simulink library "tqd"  (R2021b)
settings: Solver=VariableStepAuto  StartTime=0.0  StopTime=10.0  RelTol=1e-3
undefined symbols (not defined in the file): ATQD_AfterTqMinGain_X_Deg, ATQD_APSCreepBaseTqD_X_kph, ATQD_APSCreepBaseTqD_Y_Deg, ATQD_APSCreepBaseTqR_X_kph, ATQD_APSCreepBaseTqR_Y_Deg, ATQD_APSCreepIterm_X_kph, ATQD_APSCreepIterm_Y_kph, ATQD_APSCreepPterm_X_kph, ATQD_APSCreepPterm_Y_kph, ATQD_APSDecReq_X_kph, ATQD_APSDecReq_Y_mps2, ATQD_APSDecReqCMD_X_kph, ATQD_APSDecReqTs_X_pct, ATQD_APSDecTimeGain_X_Deg, ATQD_APSDecTimeGain_Y_s, ATQD_APSReqLowSpd_X_Deg, ATQD_AutoHoldReleaseBPS_X_Deg, ATQD_AWDLoadTrqnsGain_X_kg, ATQD_AWDLoadTrqnsGain_Y_pct, ATQD_BOSEnBPSPosn_X_kph, ATQD_BOSMap_X_rpm, ATQD_BOSMap_Y_pct, ATQD_CreepBaseTqD_X_kph, ATQD_CreepBaseTqD_Y_Deg, ATQD_CreepBaseTqR_X_kph, ATQD_CreepBaseTqR_Y_Deg, ATQD_CreepBPSDisPosn_X_Deg, ATQD_CreepBPSDisPosnR_X_Deg, ATQD_CreepBPSEnPosn_X_Deg, ATQD_CreepBPSEnPosnR_X_Deg, ATQD_CreepDeltaTq_X_kph, ATQD_CreepIterm_X_kph, ATQD_CreepIterm_Y_kph, ATQD_CreepItermMaxLimit_X_pct, ATQD_CreepPreloadTime_X_kph, ATQD_CreepPreloadTq_X_kph, ATQD_CreepPreloadTq_Y_s, ATQD_CreepProtTq_X_Deg, ATQD_CreepPterm_X_kph, ATQD_CreepPterm_Y_kph, ATQD_CreepRrTqSpRat_X_rpm, ATQD_CreepRrTqSpRat_Y_Nm, ATQD_CreepTargetSpdD_X_pct, ATQD_CreepTargetSpdR_X_pct, ATQD_ECOTqMapD_X_rpm, ATQD_ECOTqMapD_Y_pct, ATQD_EMTqMapD_X_rpm, ATQD_EMTqMapD_Y_pct, ATQD_EOPDTqMapDCon_X_rpm, ATQD_EOPDTqMapDCon_Y_Deg, ATQD_EscapeModePedTq_X_pct, ATQD_EscapeModePedTq_Y_rpm, ATQD_EscapeModePedTqFr_X_pct, ATQD_EscapeModePedTqFr_Y_rpm, ATQD_EstInitVehWeight_X_c, ATQD_FAfterTqCMDGain_X_rpm, ATQD_FAfterTqCMDGain_Y_pct, ATQD_FrLossMAPLowV_X_rpm, ATQD_FrLossMAPLowV_Y_Nm, ATQD_FrMotActReduce_X_rpm ... (+772)
libraries: simulink x211, hcu_lib x179, tqr x3
(part 15 of 28)

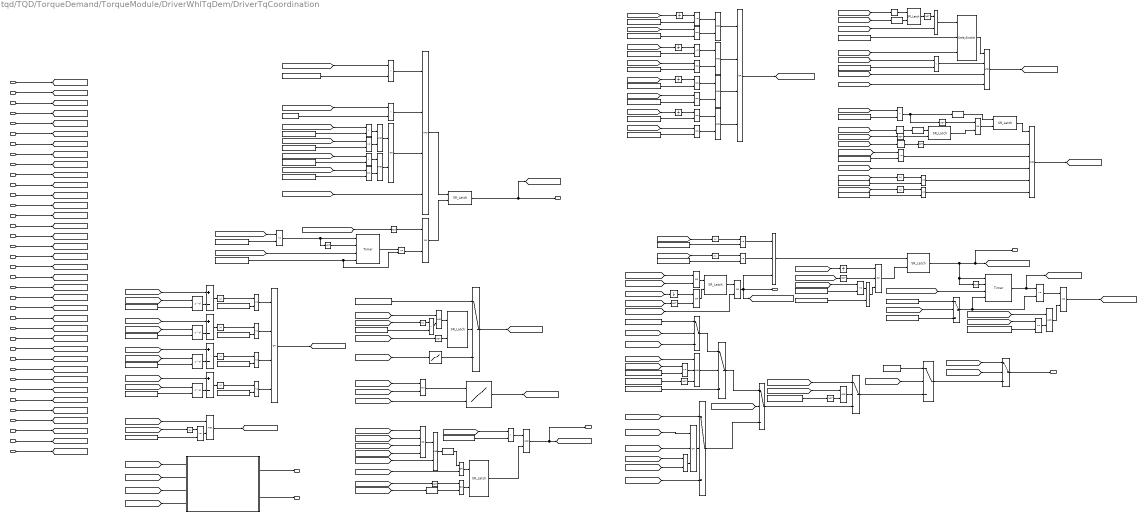
== system tqd/TQD/TorqueDemand/TorqueModule/DriverWhlTqDem/DriverTqCoordination ==
  VTQD_PedalMapWhlTq_Nm : Inport
  VTQD_CreepPrLoadEnable_flg : Inport  Port=2
  VTQD_CreepWhlTqDem_Nm : Inport  Port=3
  VTQD_BOSEnable_flg : Inport  Port=4
  VTQD_BOSTq_Nm : Inport  Port=5
  VVMC_LongAcc_Gps : Inport  Port=6
  VINP_VehSpeed_kph : Inport  Port=7
  VTQD_BrkSwSta_flg : Inport  Port=8
  VTQD_ActBPSPosn_pct : Inport  Port=9
  VTQD_LowIdleAccPedal_flg : Inport  Port=10
  VTQD_GearActualPosn_enum : Inport  Port=11
  task_time_s : Inport  Port=12
  VINP_FrEDURealTMTq_Nm : Inport  Port=13
  VINP_RrEDURealTMTq_Nm : Inport  Port=14
  VVMC_APSActive_flg : Inport  Port=15
  VVMC_ADASActive_flg : Inport  Port=16
  VINP_ACCVehHoldReq_flg : Inport  Port=17
  VTQD_CreepProtTqEn_flg : Inport  Port=18
  VTQD_TqTargetShaftSpd_rpm : Inport  Port=19
  VTQD_VehActSpd_kph : Inport  Port=20
  VTQD_APSReqTimer_s : Inport  Port=21
  VTQD_CreepEnable_flg : Inport  Port=22
  VTQR_RShaftSpdTqLimLow_flg : Inport  Port=23
  VTQR_RTimerTqLimLow_flg : Inport  Port=24
  VTQR_FShaftSpdTqLimLow_flg : Inport  Port=25
  VTQR_FTimerTqLimLow_flg : Inport  Port=26
  VTQD_ActAPSPosn_pct : Inport  Port=27
  VTQD_IVIRockModeEn_flg : Inport  Port=28
  VINP_LFRawWhlSpeed_kph : Inport  Port=29
  VINP_LRRawWhlSpeed_kph : Inport  Port=30
  VINP_RFRawWhlSpeed_kph : Inport  Port=31
  VINP_RRRawWhlSpeed_kph : Inport  Port=32
  VTQD_FrShaftSpd_rpm : Inport  Port=33
  VTQD_RrShaftSpd_rpm : Inport  Port=34
  VINP_ADASAEBSta_enum : Inport  Port=35
  VTQD_ActWhlSkipSta_enum : Inport  Port=36
  VDDM_VehMalfunLevel_enum : Inport  Port=37
  AND : Logic  Inputs=3  AllPortsSameDT=off  OutDataTypeStr=boolean
  AND{1..3,7..17} (14 alike) : Logic  AllPortsSameDT=off  OutDataTypeStr=boolean
  AND4 : Logic  Inputs=6  AllPortsSameDT=off  OutDataTypeStr=boolean
  AND5 : Logic  Inputs=4  AllPortsSameDT=off  OutDataTypeStr=boolean
  AND6 : Logic  Inputs=4  AllPortsSameDT=off  OutDataTypeStr=boolean
  Abs{,1..9} (10 alike) : Abs
  Add{,1..3} (4 alike) : Sum  Inputs=+-
  Constant : Constant  Value=KTQD_LoSpdCtrlBrkPos_pct
  Constant1 : Constant  Value=KTQD_RrPreLoadBoundary_Nm
  Constant{2,10,15,17} (4 alike) : Constant  Value=ZERO_FLOAT
  Constant11 : Constant  Value=KTQD_ADASHoldPreLoadspd_kph
  Constant12 : Constant  Value=KTQD_ADASHoldDelayEnTime_s
  Constant13 : Constant  Value=KTQD_EmergBrkSpd_kph
  Constant14 : Constant  Value=KTQD_EmergBrkLongAccel_Gps
  Constant16 : Constant  Value=KTQD_PreLoadTqHold_rpm
  Constant18 : Constant  Value=KTQD_OPDHoldPreLoadTime_s
  Constant19 : Constant  Value=KTQD_PreLoad_Holdtime_s
  Constant20 : Constant  Value=KTQD_APSZeroSpd_kph
  Constant21 : Constant  Value=ENUM_GEARACTUALPOSN_D
  Constant22 : Constant  Value=ENUM_GEARACTUALPOSN_D
  Constant{4,6,23..24} (4 alike) : Constant  Value=ENUM_GEARACTUALPOSN_R
  Constant25 : Constant  Value=KTQD_LoSPdBrkRlsTime_s
  Constant26 : Constant  Value=KTQD_LoSpdBrkRlsSpd_kph
  Constant27 : Constant  Value=KTQD_OPDHoldPreLoadBound_Nm
  Constant28 : Constant  Value=KTQD_OPDHoldPreLoadBound_Nm
  Constant29 : Constant  Value=KTQD_PreLoadDisSpd_kph
  Constant3 : Constant  Value=KTQD_RrPreLoadBoundary_Nm
  Constant{30,32,34,36} (4 alike) : Constant  Value=KTQD_EscModeWhlSpdDely_cnt
  Constant{31,33,35,37} (4 alike) : Constant  Value=KTQD_EscModeTqLimSpdDev_kph
  Constant38 : Constant  Value=KTQD_EscModeTqLimAccCon_Gps
  Constant39 : Constant  Value=KTQD_ESCModeTqCtrlSW_flg
  Constant40 : Constant  Value=ENUM_ADASAEBSTA_ACTIVE
  Constant41 : Constant  Value=KTQD_AEBEmergBrkSpd_kph
  Constant42 : Constant  Value=KTQD_APSPreLoadHoldtime_s
  Constant43 : Constant  Value=KTQD_RockModeWhlSkipSta_enum
  Constant44 : Constant  Value=KTQD_NewPrelaodSW_flg
  Constant45 : Constant  Value=ENUM_VEHMALFUNLEVEL_LEVEL3
  Constant5 : Constant  Value=ENUM_GEARACTUALPOSN_N
  Constant7 : Constant  Value=ENUM_GEARACTUALPOSN_P
  Constant8 : Constant  Value=ENUM_GEARACTUALPOSN_P
  Constant9 : Constant  Value=KTQD_PreLoadTq_Nm
  Constant96 : Constant  Value=KTQD_FailsafeActiveSW_flg
  Delay : Delay  DelayLength=1
  Delay1 : Delay  DelayLength=1
  Delay2 : Delay  DelayLength=1
  Delay{3..6} (4 alike) : Delay  DelayLengthSource=Input port
      settings: InputPortMap=u0,p1
  DelayEnable : hcu_lib/Basic_Blocks/DelayEnable
  Detect Change : simulink/Logic and Bit Operations/Detect Change  vinit=0  OutDataTypeStr=boolean
  Detect Decrease : simulink/Logic and Bit Operations/Detect Decrease  vinit=0.0  OutDataTypeStr=boolean
  Detect Increase : simulink/Logic and Bit Operations/Detect Increase  vinit=0.0  OutDataTypeStr=boolean
  Detect Increase1 : simulink/Logic and Bit Operations/Detect Increase  vinit=0.0  OutDataTypeStr=boolean
  Detect Increase2 : simulink/Logic and Bit Operations/Detect Increase  vinit=0.0  OutDataTypeStr=boolean
  Equal{1..4,6,8} (6 alike) : RelationalOperator  Operator===  OutDataTypeStr=boolean  RndMeth=Simplest
  Equal5 : RelationalOperator  Operator=~=  OutDataTypeStr=boolean  RndMeth=Simplest
  Equal7 : RelationalOperator  Operator=~=  OutDataTypeStr=boolean  RndMeth=Simplest
  Equal9 : RelationalOperator  Operator=~=  OutDataTypeStr=boolean  RndMeth=Simplest
  GreaterThan : RelationalOperator  OutDataTypeStr=boolean  RndMeth=Simplest
  Logical Operator : Logic  Inputs=3  AllPortsSameDT=off  OutDataTypeStr=boolean
  Logical Operator13 : Logic  AllPortsSameDT=off  OutDataTypeStr=boolean
  MTQD_EscapeModePedTq_Z_Nm : Lookup_n-D  BreakpointsForDimension1=ATQD_EscapeModePedTq_Y_rpm  BreakpointsForDimension2=ATQD_EscapeModePedTq_X_pct  Table=MTQD_EscapeModePedTq_Z_Nm  InternalRulePriority=Speed  RndMeth=Simplest  InputSameDT=on
      settings: InputPortMap=u0,u1
  MTQD_PreLoadTq_Y_Nm : Lookup_n-D  NumberOfTableDimensions=1  BreakpointsForDimension1=ATQD_PreLoadTq_X_s  Table=MTQD_PreLoadTq_Y_Nm  ExtrapMethod=Clip  InternalRulePriority=Speed  RndMeth=Simplest  InputSameDT=on
  Max : MinMax  Function=max  Inputs=2
  NOT{,1..12} (13 alike) : Logic  Operator=NOT  AllPortsSameDT=off  OutDataTypeStr=boolean
  New Preload Torque : Subsystem
  OR : Logic  Operator=OR  Inputs=3  AllPortsSameDT=off  OutDataTypeStr=boolean
  OR{2,4..8,10,12..13} (9 alike) : Logic  Operator=OR  AllPortsSameDT=off  OutDataTypeStr=boolean
  OR11 : Logic  Operator=OR  Inputs=4  AllPortsSameDT=off  OutDataTypeStr=boolean
  OR14 : Logic  Operator=OR  Inputs=3  AllPortsSameDT=off  OutDataTypeStr=boolean
  OR3 : Logic  Operator=OR  Inputs=4  AllPortsSameDT=off  OutDataTypeStr=boolean
  OR9 : Logic  Operator=OR  Inputs=4  AllPortsSameDT=off  OutDataTypeStr=boolean
  Relational Operator{,7,15..18,23} (7 alike) : RelationalOperator  OutDataTypeStr=boolean  RndMeth=Simplest
  Relational Operator{1..2,6,11..14,19} (8 alike) : RelationalOperator  Operator=<=  OutDataTypeStr=boolean  RndMeth=Simplest
  Relational Operator{3,8..10,21} (5 alike) : RelationalOperator  Operator=<  OutDataTypeStr=boolean  RndMeth=Simplest
  Relational Operator20 : RelationalOperator  Operator===  OutDataTypeStr=boolean  RndMeth=Simplest
  Relational Operator22 : RelationalOperator  Operator=>  OutDataTypeStr=boolean  RndMeth=Simplest
  Relational Operator4 : RelationalOperator  Operator=>  OutDataTypeStr=boolean  RndMeth=Simplest
  Relational Operator5 : RelationalOperator  Operator=>  OutDataTypeStr=boolean  RndMeth=Simplest
  SR_Latch{,1..7} (8 alike) : hcu_lib/Basic_Blocks/SR_Latch
  Switch{,1..4} (5 alike) : Switch  Criteria=u2 ~= 0
      Switch1 settings: AttributesFormatString=<%<Criteria>>
      Switch2 settings: AttributesFormatString=<%<Criteria>>
  Switch{5..8} (4 alike) : Switch  Criteria=u2 > Threshold
  Timer : hcu_lib/Basic_Blocks/Timer
  Timer1 : hcu_lib/Basic_Blocks/Timer
  Unit Delay{1..6} (6 alike) : UnitDelay  SampleTime=-1  HasFrameUpgradeWarning=on
  VTQD_DriverWhlTqDem_Nm : Outport
  VTQD_LoSpdBrkCtrl_flg : Outport  Port=2
  VTQD_PreLoadHold_flg : Outport  Port=3
  VTQD_PreLoadPreEn_flg : Outport  Port=4
  VTQD_EscapModeTqLim_flg : Outport  Port=5
  VTQD_FrPreloadTq_Nm : Outport  Port=6
  VTQD_RrPreloadTq_Nm : Outport  Port=7
  wires:
  VTQD_PedalMapWhlTq_Nm/1 -> [VTQD_PedalMapWhlTq_Nm]
  VTQD_CreepPrLoadEnable_flg/1 -> [VTQD_CreepPrLoadEnable_flg]
  VTQD_CreepWhlTqDem_Nm/1 -> [VTQD_CreepWhlTqDem_Nm]
  VTQD_BOSEnable_flg/1 -> [VTQD_BOSEnable_flg]
  VTQD_BOSTq_Nm/1 -> [VTQD_BOSTq_Nm]
  [VTQD_BOSEnable_flg] -> Switch1/2
  [VTQD_PedalMapWhlTq_Nm] -> Switch2/3
  [VTQD_CreepWhlTqDem_Nm] -> Switch2/1
  [VTQD_ActBPSPosn_pct] -> Relational Operator/1
  Constant/1 -> Relational Operator/2
  SR_Latch/1 -> [VTQD_LoSpdBrkCtrl_flg], VTQD_LoSpdBrkCtrl_flg/1  "VTQD_LoSpdBrkCtrl_flg"
  Constant10/1 -> Switch/1
  Switch1/1 -> VTQD_DriverWhlTqDem_Nm/1  "VTQD_DriverWhlTqDem_Nm"
  Switch/1 -> Switch1/3
  [VTQD_LowIdleAccPedal_flg] -> NOT/1
  [VTQD_VehActSpd_kph] -> Relational Operator6/1
  Constant26/1 -> Relational Operator6/2
  Relational Operator6/1 -> Timer/1, NOT1/1
  Timer/1 -> Relational Operator7/1
  NOT/1 -> OR2/1
  Relational Operator7/1 -> OR2/2
  OR2/1 -> SR_Latch/2  "VTQD_LoBrkCtrlReset_flg"
  NOT1/1 -> Timer/2
  Constant13/1 -> Relational Operator10/2
  [VINP_VehSpeed_kph] -> Relational Operator10/1
  Constant15/1 -> Relational Operator9/2
  Constant14/1 -> Relational Operator8/2
  [VVMC_LongAcc_Gps] -> Relational Operator8/1
  Relational Operator9/1 -> AND6/2
  Relational Operator8/1 -> AND6/1
  [task_time_s] -> Timer/3
  VVMC_LongAcc_Gps/1 -> [VVMC_LongAcc_Gps]
  VINP_VehSpeed_kph/1 -> [VINP_VehSpeed_kph]
  VTQD_BrkSwSta_flg/1 -> [VTQD_BrkSwSta_flg]
  VTQD_ActBPSPosn_pct/1 -> [VTQD_ActBPSPosn_pct]
  VTQD_LowIdleAccPedal_flg/1 -> [VTQD_LowIdleAccPedal_flg]
  VTQD_GearActualPosn_enum/1 -> [VTQD_GearActualPosn_enum]
  task_time_s/1 -> [task_time_s]
  Constant25/1 -> Relational Operator7/2, Timer/4
  AND6/1 -> SR_Latch/1  "VTQD_TestLoSpdBrkCtrl_flg"
  Timer1/1 -> [VTQD_PreLoadHoldtime_s], GreaterThan/1  "VTQD_PreLoadHoldtime_s"
  [VTQD_PreLoadPreEn_flg] -> Switch4/2
  [VTQD_HoldtimeEnd_flg] -> Unit Delay4/1
  [task_time_s] -> Timer1/3
  Unit Delay2/1 -> Equal5/1
  [VTQD_GearActualPosn_enum] -> Unit Delay2/1
  Constant23/1 -> Equal7/2
  [VTQD_GearActualPosn_enum] -> Equal8/1
  Equal5/1 -> AND8/1
  AND9/1 -> OR3/2
  Constant21/1 -> Equal5/2
  Constant24/1 -> Equal8/2
  Unit Delay3/1 -> Equal7/1
  Constant22/1 -> Equal6/2
  AND8/1 -> OR3/1
  [VTQD_GearActualPosn_enum] -> Unit Delay3/1
  [VTQD_GearActualPosn_enum] -> Equal6/1
  Equal6/1 -> AND8/2
  Equal8/1 -> AND9/2
  OR3/1 -> [VTQD_ShiftPreload_flg]  "VTQD_ShiftPreload_flg"
  Equal7/1 -> AND9/1
  NOT2/1 -> Timer1/2
  Unit Delay4/1 -> OR4/1
  OR4/1 -> SR_Latch1/2
  Switch2/1 -> Switch4/3
  [VTQD_LowIdleAccPedal_flg] -> NOT3/1
  NOT3/1 -> OR4/2
  [VTQD_LoSpdBrkCtrl_flg] -> Switch/2
  VINP_FrEDURealTMTq_Nm/1 -> [VINP_FrEDURealTMTq_Nm]
  VINP_RrEDURealTMTq_Nm/1 -> [VINP_RrEDURealTMTq_Nm]
  [VTQD_GearActualPosn_enum] -> Equal2/1
  Constant5/1 -> Equal2/2
  Equal2/1 -> AND1/2
  Equal1/1 -> AND1/1
  Constant4/1 -> Equal1/2
  AND1/1 -> OR3/3
  [VTQD_GearActualPosn_enum] -> Unit Delay1/1
  Unit Delay1/1 -> Equal1/1
  Constant3/1 -> Relational Operator2/2
  Relational Operator2/1 -> AND/1
  Constant1/1 -> Relational Operator1/2
  Abs1/1 -> Relational Operator2/1
  Relational Operator1/1 -> AND/2
  Abs/1 -> Relational Operator1/1
  [VINP_RrEDURealTMTq_Nm] -> Abs/1
  [VINP_FrEDURealTMTq_Nm] -> Abs1/1
  OR5/1 -> AND/3, VTQD_PreLoadPreEn_flg/1, [VTQD_PreLoadPreEn_flg]  "VTQD_PreLoadPreEn_flg"
  Switch3/1 -> Switch4/1
  Constant2/1 -> Switch3/3
  Unit Delay5/1 -> Equal3/1
  [VTQD_GearActualPosn_enum] -> Unit Delay5/1
  Constant6/1 -> Equal3/2
  Equal3/1 -> AND2/1
  Equal4/1 -> AND2/2
  Constant7/1 -> Equal4/2
  [VTQD_GearActualPosn_enum] -> Equal4/1
  AND2/1 -> OR3/4
  AND/1 -> SR_Latch2/1
  NOT4/1 -> OR14/2
  [VTQD_LowIdleAccPedal_flg] -> NOT4/1
  Unit Delay6/1 -> OR14/1
  [VTQD_HoldtimeEnd_flg] -> Unit Delay6/1
  [VTQD_GearActualPosn_enum] -> Equal9/1
  Constant8/1 -> Equal9/2
  Logical Operator/1 -> Switch3/2
  [VTQD_PreLoadHold_flg] -> Logical Operator/1
  Equal9/1 -> Logical Operator/2
  SR_Latch2/1 -> VTQD_PreLoadHold_flg/1, [VTQD_PreLoadHold_flg], NOT2/1, Timer1/1  "VTQD_PreLoadHold_flg"
  Constant12/1 -> DelayEnable/2
  Relational Operator3/1 -> AND5/2
  Constant11/1 -> Relational Operator3/2
  AND5/1 -> [VTQD_ADASPreLoadEn_flg]  "VTQD_ADASPreLoadEn_flg"
  AND7/1 -> DelayEnable/1  "VTQD_ADASPreLoadHold_flg"
  [VVMC_ADASActive_flg] -> AND5/3
  [VINP_ACCVehHoldReq_flg] -> Detect Increase/1
  Delay/1 -> SR_Latch3/1
  DelayEnable/1 -> AND5/1
  [VTQD_HoldtimeEnd_flg] -> Delay/1
  SR_Latch3/1 -> NOT5/1
  [VINP_ACCVehHoldReq_flg] -> AND7/2
  Detect Increase/1 -> SR_Latch3/2
  [task_time_s] -> DelayEnable/3  "task_time_s"
  [VINP_VehSpeed_kph] -> Relational Operator3/1
  NOT5/1 -> AND7/1
  Constant9/1 -> Switch5/1
  [VVMC_APSActive_flg] -> Switch5/2
  Switch5/1 -> Switch3/1
  [VVMC_APSActive_flg] -> OR/2
  OR/1 -> Switch2/2
  [VTQD_CreepPrLoadEnable_flg] -> OR/1
  [VTQD_ADASPreLoadEn_flg] -> OR5/2
  SR_Latch1/1 -> OR5/1
  VVMC_APSActive_flg/1 -> [VVMC_APSActive_flg]
  VVMC_ADASActive_flg/1 -> [VVMC_ADASActive_flg]
  VINP_ACCVehHoldReq_flg/1 -> [VINP_ACCVehHoldReq_flg]
  VTQD_CreepProtTqEn_flg/1 -> [VTQD_CreepProtTqEn_flg]
  [VTQD_CreepProtTqEn_flg] -> AND10/1
  [VTQD_LowIdleAccPedal_flg] -> AND10/2
  AND10/1 -> OR/3
  [VTQD_LowIdleAccPedal_flg] -> AND5/4
  [VTQD_PreLoadHold_flg] -> AND3/1
  Constant17/1 -> Switch6/1
  Abs2/1 -> Relational Operator4/1
  [VTQD_PreLoadHold_flg] -> NOT6/1
  [VTQD_TqTargetShaftSpd_rpm] -> Abs2/1
  Constant16/1 -> Relational Operator4/2
  NOT6/1 -> SR_Latch4/2
  Switch6/1 -> [VTQD_PreloadTq_Nm]  "VTQD_PreloadTq_Nm"
  SR_Latch4/1 -> Switch6/2
  MTQD_PreLoadTq_Y_Nm/1 -> Switch6/3
  Relational Operator4/1 -> AND3/2
  AND3/1 -> SR_Latch4/1
  [VTQD_PreLoadHoldtime_s] -> MTQD_PreLoadTq_Y_Nm/1
  [VTQD_PreloadTq_Nm] -> Switch5/3
  VTQD_TqTargetShaftSpd_rpm/1 -> [VTQD_TqTargetShaftSpd_rpm]
  [VTQD_BOSTq_Nm] -> Switch1/1
  VTQD_VehActSpd_kph/1 -> [VTQD_VehActSpd_kph]
  [VTQD_APSReqTimer_s] -> Relational Operator5/1
  Constant18/1 -> Relational Operator5/2
  Detect Increase1/1 -> SR_Latch5/1
  Relational Operator5/1 -> Detect Increase1/1, NOT8/1
  SR_Latch5/1 -> AND4/1
  AND4/1 -> [VTQD_OPDHoldPreLoadEn_flg]  "VTQD_OPDHoldPreLoadEn_flg"
  VTQD_APSReqTimer_s/1 -> [VTQD_APSReqTimer_s]
  VTQD_CreepEnable_flg/1 -> [VTQD_CreepEnable_flg]
  [VINP_VehSpeed_kph] -> Relational Operator11/1
  Constant20/1 -> Relational Operator11/2
  OR6/1 -> SR_Latch5/2
  NOT8/1 -> OR6/1
  NOT7/1 -> AND4/2
  Relational Operator11/1 -> AND4/3
  Delay2/1 -> NOT7/1
  [VTQD_CreepEnable_flg] -> Delay2/1
  Detect Increase2/1 -> SR_Latch6/1
  NOT9/1 -> SR_Latch6/2
  [VTQD_LowIdleAccPedal_flg] -> NOT9/1
  SR_Latch6/1 -> OR6/2  "VTQD_PreLoadHoldtimeEnd_flg"
  Delay1/1 -> Detect Increase2/1
  [VTQD_HoldtimeEnd_flg] -> Delay1/1
  [VTQD_LowIdleAccPedal_flg] -> AND4/4
  Abs4/1 -> Relational Operator13/1
  Relational Operator12/1 -> AND4/6
  Constant28/1 -> Relational Operator13/2
  [VINP_FrEDURealTMTq_Nm] -> Abs4/1
  Relational Operator13/1 -> AND4/5
  Abs3/1 -> Relational Operator12/1
  [VINP_RrEDURealTMTq_Nm] -> Abs3/1
  Constant27/1 -> Relational Operator12/2
  [VVMC_LongAcc_Gps] -> Relational Operator9/1
  OR7/1 -> SR_Latch1/1
  [VTQD_ShiftPreload_flg] -> OR7/2
  [VTQD_OPDHoldPreLoadEn_flg] -> OR7/1
  [VTQD_VehActSpd_kph] -> Relational Operator14/1
  [VTQD_PreLoadHold_flg] -> AND11/1
  Constant29/1 -> Relational Operator14/2
  Relational Operator14/1 -> AND11/2
  AND11/1 -> OR8/2
  GreaterThan/1 -> OR8/1
  OR8/1 -> [VTQD_HoldtimeEnd_flg]  "VTQD_HoldtimeEnd_flg"
  VTQR_RShaftSpdTqLimLow_flg/1 -> [VTQR_RShaftSpdTqLimLow_flg]
  VTQR_RTimerTqLimLow_flg/1 -> [VTQR_RTimerTqLimLow_flg]
  VTQR_FShaftSpdTqLimLow_flg/1 -> [VTQR_FShaftSpdTqLimLow_flg]
  VTQD_IVIRockModeEn_flg/1 -> [VTQD_IVIRockModeEn_flg]
  VTQD_ActAPSPosn_pct/1 -> [VTQD_ActAPSPosn_pct]
  VTQR_FTimerTqLimLow_flg/1 -> [VTQR_FTimerTqLimLow_flg]
  MTQD_EscapeModePedTq_Z_Nm/1 -> [VTQD_EscapeModePedTq_Nm]  "VTQD_EscapeModePedTq_Nm"
  [VTQR_FTimerTqLimLow_flg] -> OR9/4
  [VTQR_FShaftSpdTqLimLow_flg] -> OR9/3
  [VTQR_RTimerTqLimLow_flg] -> OR9/2
  [VTQR_RShaftSpdTqLimLow_flg] -> OR9/1
  OR9/1 -> AND12/1
  [VTQD_IVIRockModeEn_flg] -> AND12/2
  OR10/1 -> SR_Latch7/2
  NOT10/1 -> OR10/1
  [VTQD_IVIRockModeEn_flg] -> NOT10/1
  Detect Change/1 -> OR10/2
  [VTQD_GearActualPosn_enum] -> Detect Change/1
  AND12/1 -> Detect Decrease/1
  Switch4/1 -> Switch7/3
  [VTQD_EscapeModePedTq_Nm] -> Switch7/1
  Switch7/1 -> Switch/3
  VINP_LRRawWhlSpeed_kph/1 -> [VINP_LRRawWhlSpeed_kph]
  VINP_RFRawWhlSpeed_kph/1 -> [VINP_RFRawWhlSpeed_kph]
  VINP_RRRawWhlSpeed_kph/1 -> [VINP_RRRawWhlSpeed_kph]
  VINP_LFRawWhlSpeed_kph/1 -> [VINP_LFRawWhlSpeed_kph]
  [VINP_LFRawWhlSpeed_kph] -> Delay3/1
  Constant30/1 -> Delay3/2
  Delay3/1 -> Add/2
  [VINP_LFRawWhlSpeed_kph] -> Add/1
  Add/1 -> Abs5/1
  Abs5/1 -> Relational Operator15/1
  Constant31/1 -> Relational Operator15/2
  Relational Operator15/1 -> OR11/1
  Constant33/1 -> Relational Operator16/2
  Abs6/1 -> Relational Operator16/1
  Add1/1 -> Abs6/1
  [VINP_LRRawWhlSpeed_kph] -> Add1/1
  Delay4/1 -> Add1/2
  Constant32/1 -> Delay4/2
  [VINP_LRRawWhlSpeed_kph] -> Delay4/1
  [VINP_RFRawWhlSpeed_kph] -> Delay5/1
  Constant34/1 -> Delay5/2
  Delay5/1 -> Add2/2
  [VINP_RFRawWhlSpeed_kph] -> Add2/1
  Add2/1 -> Abs7/1
  Abs7/1 -> Relational Operator17/1
  Constant35/1 -> Relational Operator17/2
  Constant37/1 -> Relational Operator18/2
  Abs8/1 -> Relational Operator18/1
  Add3/1 -> Abs8/1
  [VINP_RRRawWhlSpeed_kph] -> Add3/1
  Delay6/1 -> Add3/2
  Constant36/1 -> Delay6/2
  [VINP_RRRawWhlSpeed_kph] -> Delay6/1
  Relational Operator16/1 -> OR11/2
  Relational Operator17/1 -> OR11/3
  Relational Operator18/1 -> OR11/4
  OR11/1 -> [VTQD_WhlQuickSkip_flg]  "VTQD_WhlQuickSkip_flg"
  OR12/1 -> SR_Latch7/1
  Detect Decrease/1 -> OR12/1
  [VTQD_WhlSpdQuickSkip_flg] -> OR12/2
  [VTQD_WhlQuickSkip_flg] -> AND13/1
  Relational Operator19/1 -> AND13/2
  [VVMC_LongAcc_Gps] -> Abs9/1
  Constant38/1 -> Relational Operator19/2
  Abs9/1 -> Relational Operator19/1
  AND13/1 -> [VTQD_WhlSpdQuickSkip_flg]  "VTQD_WhlSpdQuickSkip_flg"
  VTQD_RrShaftSpd_rpm/1 -> [VTQD_RrShaftSpd_rpm]
  VTQD_FrShaftSpd_rpm/1 -> [VTQD_FrShaftSpd_rpm]
  [VTQD_RrShaftSpd_rpm] -> Max/2
  [VTQD_FrShaftSpd_rpm] -> Max/1
  Max/1 -> MTQD_EscapeModePedTq_Z_Nm/1  "VTQD_MaxShaftSpd_rpm"
  [VTQD_ActAPSPosn_pct] -> MTQD_EscapeModePedTq_Z_Nm/2
  AND14/1 -> Switch7/2
  [VTQD_EscapModeTqLim_flg] -> AND14/1
  NOT11/1 -> AND14/2
  Constant39/1 -> NOT11/1
  [VTQD_BrkSwSta_flg] -> AND6/4
  OR13/1 -> AND6/3
  Relational Operator10/1 -> AND16/1
  Relational Operator/1 -> AND16/2
  AND16/1 -> OR13/1
  Relational Operator20/1 -> AND15/2
  Relational Operator21/1 -> AND15/1
  [VINP_VehSpeed_kph] -> Relational Operator21/1
  Constant41/1 -> Relational Operator21/2
  Constant40/1 -> Relational Operator20/2
  [VINP_ADASAEBSta_enum] -> Relational Operator20/1
  AND15/1 -> OR13/2
  VINP_ADASAEBSta_enum/1 -> [VINP_ADASAEBSta_enum]
  Constant19/1 -> Switch8/3
  Switch8/1 -> GreaterThan/2, Timer1/4
  [VVMC_APSActive_flg] -> Switch8/2
  Constant42/1 -> Switch8/1
  VTQD_ActWhlSkipSta_enum/1 -> [VTQD_ActWhlSkipSta_enum]
  AND17/1 -> [VTQD_EscapModeTqLim_flg], VTQD_EscapModeTqLim_flg/1  "VTQD_EscapModeTqLim_flg"
  SR_Latch7/1 -> AND17/2
  [VTQD_ActWhlSkipSta_enum] -> Relational Operator22/1
  Constant43/1 -> Relational Operator22/2
  Relational Operator22/1 -> AND17/1
  [VTQD_PreLoadHold_flg] -> New Preload Torque/1(VTQD_PreLoadHold_flg)
  [VTQD_PreLoadHoldtime_s] -> New Preload Torque/2(VTQD_PreLoadHoldtime_s)
  [VTQD_FrShaftSpd_rpm] -> New Preload Torque/3(VTQD_FrShaftSpd_rpm)
  [VTQD_RrShaftSpd_rpm] -> New Preload Torque/4(VTQD_RrShaftSpd_rpm)
  New Preload Torque/1(VTQD_FrPreloadTq_Nm) -> VTQD_FrPreloadTq_Nm/1
  New Preload Torque/2(VTQD_RrPreloadTq_Nm) -> VTQD_RrPreloadTq_Nm/1
  Constant44/1 -> NOT12/1
  NOT12/1 -> Logical Operator/3
  VDDM_VehMalfunLevel_enum/1 -> [VDDM_VehMalfunLevel_enum]
  OR14/1 -> SR_Latch2/2
  Constant96/1 -> Logical Operator13/2
  Relational Operator23/1 -> Logical Operator13/1
  [VDDM_VehMalfunLevel_enum] -> Relational Operator23/1
  Constant45/1 -> Relational Operator23/2
  Logical Operator13/1 -> OR14/3

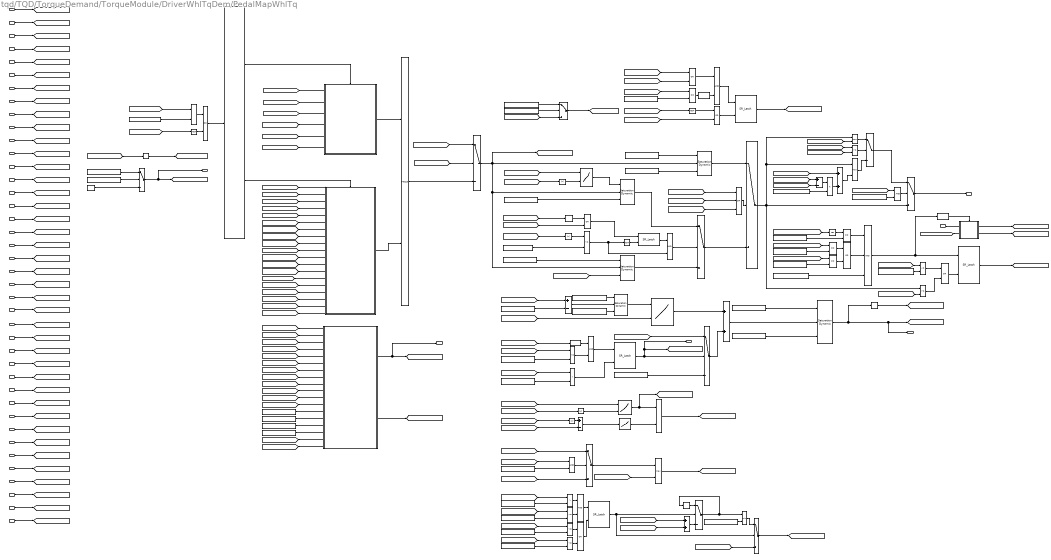
== system tqd/TQD/TorqueDemand/TorqueModule/DriverWhlTqDem/PedalMapWhlTq ==
  VTQD_GearActualPosn_enum : Inport
  VTQD_ActAPSPosn_pct : Inport  Port=2
  VTQD_TqTargetShaftSpd_rpm : Inport  Port=3
  VTQD_LimpHomeAct_flg : Inport  Port=4
  VTQD_EVDriveMode_enum : Inport  Port=5
  VTQD_RegenMode_enum : Inport  Port=6
  VTQD_RollRegenEnable_flg : Inport  Port=7
  VTQD_RollingShaftSpd_rpm : Inport  Port=8
  VTQD_RollRegenDisableReq_flg : Inport  Port=9
  VINP_HSAActive_flg : Inport  Port=10
  VVMC_ADASActive_flg : Inport  Port=11
  VVMC_ActMaxSlideRate_pct : Inport  Port=12
  VVMC_EstSlope_Deg : Inport  Port=13
  VVMC_LongAcc_Gps : Inport  Port=14
  VTQD_SysMode_enum : Inport  Port=15
  VPMM_PwrSta_enum : Inport  Port=16
  VINP_SWCResUpSta_flg : Inport  Port=17
  task_time_s : Inport  Port=18
  VINP_VehSpeed_kph : Inport  Port=19
  VTQD_CreepPrLoadEnable_flg : Inport  Port=20
  VINP_BrkPedalPos_pct : Inport  Port=21
  VTQR_NoABSREDUWhlTqReq_Nm : Inport  Port=22
  VTQR_NoABSFEDUWhlTqReq_Nm : Inport  Port=23
  VINP_FrPTCSActive_flg : Inport  Port=24
  VINP_RrPTCSActive_flg : Inport  Port=25
  VINP_ADASACCSta_enum : Inport  Port=26
  VTQD_LowIdleAccPedal_flg : Inport  Port=27
  VTQD_BrkSwSta_flg : Inport  Port=28
  VTQD_OPDHoldEnRel_flg : Inport  Port=29
  VINP_SASAngle_Deg : Inport  Port=30
  VINP_YawRate_degps : Inport  Port=31
  VVMC_ActStESCYaw_degps : Inport  Port=32
  VTQD_APSReqTimer_s : Inport  Port=33
  VVMC_LastADASWhlTqReq_Nm : Inport  Port=34
  VTQD_OPDHoldActRelTq_Nm : Inport  Port=35
  VTQD_VehActSpd_kph : Inport  Port=36
  VINP_IVISnowModeCmd_flg : Inport  Port=37
  VTQD_IVIRockModeEn_flg : Inport  Port=38
  VTQD_CreepEnable_flg : Inport  Port=39
  VINP_SWC2RCustomizeSta_flg : Inport  Port=40
  VDDM_VehMalfunLevel_enum : Inport  Port=41
  AND{,1..4,6} (6 alike) : Logic  AllPortsSameDT=off  OutDataTypeStr=boolean
  AND5 : Logic  Inputs=3  AllPortsSameDT=off  OutDataTypeStr=boolean
  AND7 : Logic  Operator=OR  AllPortsSameDT=off  OutDataTypeStr=boolean
  Abs{,1..3} (4 alike) : Abs
  Add : Sum  Inputs=+-
  Add1 : Sum
  Add13 : Sum  Inputs=+-
  Add2 : Sum
  Add3 : Sum
  Add4 : Sum  Inputs=+-
  Constant1 : Constant  Value=KTQD_RgnEnLatchSpd_kph
  Constant10 : Constant  Value=KTQD_ClimbMin_rpm
  Constant11 : Constant  Value=KTQD_PedalMapRDCUpLim_Nm
  Constant12 : Constant  Value=KTQD_PedalMapRDCLowLim_Nm
  Constant13 : Constant  Value=KTQD_GRADE_Deg_ovrdval
  Constant14 : Constant  Value=KTQD_PedalMapRDCUpLim_Nm
  Constant15 : Constant  Value=KTQD_TargetSlideRate_pct
  Constant16 : Constant  Value=KTQD_SlideRateDevUpLim_pct
  Constant17 : Constant  Value=KTQD_SlideRateDevLowLim_pct
  Constant18 : Constant  Value=KTQD_PedalMapRDCLowLim_Nm
  Constant19 : Constant  Value=KTQD_SlideRegEnLimitTq_Nm
  Constant2 : Constant  Value=TRUE
  Constant20 : Constant  Value=KTQD_SlideRegEnLimitTq_Nm
  Constant21 : Constant  Value=KTQD_OrigPedTqLowLimSW_flg
  Constant22 : Constant  Value=KTQD_PedalMapRDCLowLim_Nm
  Constant23 : Constant  Value=KTQD_SlideRegenLowLim_Nm
  Constant24 : Constant  Value=KTQD_RgnEnLatchBrkPos_pct
  Constant25 : Constant  Value=ENUM_ADASACCSTA_SHUTOFF
  Constant26 : Constant  Value=KTQD_RgnEnLatchBrkPos_pct
  Constant27 : Constant  Value=KTQD_RgnEnLatchSlope_Deg
  Constant28 : Constant  Value=ZERO_FLOAT
  Constant29 : Constant  Value=ENUM_ADASACCSTA_STANDBY
  Constant3 : Constant  Value=KTQD_EVDriveModeValid_ovrdflg
  Constant30 : Constant  Value=ENUM_ADASACCSTA_OFF
  Constant31 : Constant  Value=KTQD_ACCOvrdCancelResPedTq_pct
  Constant32 : Constant  Value=KTQD_ACCOvrdCancelTqCtrl_flg
  Constant33 : Constant  Value=KVMC_ACCOvrdTestSW_flg
  Constant34 : Constant  Value=KTQD_IVICreepOnSW_flg
  Constant4 : Constant  Value=KTQD_GRADE_Deg_ovrdflg
  Constant5 : Constant  Value=KTQD_PedalMapClimbLowLim_Nm
  Constant6 : Constant  Value=KTQD_EVDriveModeValid_ovrdval
  Constant69 : Constant  Value=KTQD_ACCOvrdCancelPedTqRat_Nm
  Constant7 : Constant  Value=KTQD_IVIPedalGRegenLim_pct
  Constant72 : Constant  Value=ENUM_ADASACCSTA_OVERRIDE
  Constant8 : Constant  Value=KTQD_SmartRegenReq_mps2
  Constant9 : Constant  Value=KTQD_IVISmartRegenSW_flg
  Constant99 : Constant  Value=KTQD_FailsafeActiveSW_flg
  Delay : Delay  DelayLength=1
  Delay1 : Delay  DelayLength=1
  Delay2 : Delay  DelayLength=1
  Detect Decrease : simulink/Logic and Bit Operations/Detect Decrease  vinit=0.0  OutDataTypeStr=boolean
  Detect Increase : simulink/Logic and Bit Operations/Detect Increase  vinit=0.0  OutDataTypeStr=boolean
  Detect Increase1 : simulink/Logic and Bit Operations/Detect Increase  vinit=0.0  OutDataTypeStr=boolean
  Divide7 : Product  Inputs=**
  Equal : RelationalOperator  Operator===  OutDataTypeStr=boolean  RndMeth=Simplest
  GearShiftCheck : If  IfExpression=u1~= 0
  LHM : Subsystem  TreatAsAtomicUnit=on
  Logical Operator : Logic  Operator=OR  AllPortsSameDT=off  OutDataTypeStr=boolean
  Logical Operator1 : Logic  Operator=NOT  AllPortsSameDT=off  OutDataTypeStr=boolean
  Logical Operator18 : Logic  AllPortsSameDT=off  OutDataTypeStr=boolean
  Logical Operator2 : Logic  Operator=OR  Inputs=3  AllPortsSameDT=off  OutDataTypeStr=boolean
  Logical Operator3 : Logic  Operator=OR  AllPortsSameDT=off  OutDataTypeStr=boolean
  MTQD_OrigPedTqLowLim_Z_Nm : Lookup_n-D  BreakpointsForDimension1=ATQD_OrigPedTqLowLim_Y_pct  BreakpointsForDimension2=ATQD_OrigPedTqLowLim_X_Deg  Table=MTQD_OrigPedTqLowLim_Z_Nm  ExtrapMethod=Clip  InternalRulePriority=Speed  RndMeth=Simplest  InputSameDT=on
      settings: InputPortMap=u0,u1
  MTQD_PedalMapClimbUpLim_Z_Nm : Lookup_n-D  BreakpointsForDimension1=ATQD_PedalMapClimbUpLim_Y_Deg  BreakpointsForDimension2=ATQD_PedalMapClimbUpLim_X_rpm  Table=MTQD_PedalMapClimbUpLim_Z_Nm  ExtrapMethod=Clip  InternalRulePriority=Speed  RndMeth=Simplest  InputSameDT=on
      settings: InputPortMap=u0,u1
  "MTQD_SlideRegenTqGain_Z_Nm " : Lookup_n-D  BreakpointsForDimension1=ATQD_SlideRegenTqGain_Y_pct  BreakpointsForDimension2=ATQD_SlideRegenTqGain_X_Gps  Table=MTQD_SlideRegenTqGain_Z_Nm  ExtrapMethod=Clip  InternalRulePriority=Speed  RndMeth=Simplest  InputSameDT=on
      settings: InputPortMap=u0,u1
  MTQD_YawTqLowLim_Y_Nm : Lookup_n-D  NumberOfTableDimensions=1  BreakpointsForDimension1=ATQD_YawTqLowLim_X_degps  Table=MTQD_YawTqLowLim_Y_Nm  ExtrapMethod=Clip  InternalRulePriority=Speed  RndMeth=Simplest  InputSameDT=on
  Max{,1..3} (4 alike) : MinMax  Function=max  Inputs=2
  Merge : Merge
  Min : MinMax  Inputs=2
  NOT : Logic  Operator=NOT  AllPortsSameDT=off  OutDataTypeStr=boolean
  NOT1 : Logic  Operator=NOT  AllPortsSameDT=off  OutDataTypeStr=boolean
  NoLHM : Subsystem  AncestorBlock=tqd0/TQD/TorqueDemand/TorqueModule/DriverWhlTqDem/PedalMapWhlTq/NoLHM  TreatAsAtomicUnit=on
  OR{,1..3} (4 alike) : Logic  Operator=OR  AllPortsSameDT=off  OutDataTypeStr=boolean
  Pedal G-Control Mode : Subsystem  AncestorBlock=tqd0/TQD/TorqueDemand/TorqueModule/DriverWhlTqDem/PedalMapWhlTq/Pedal G-Control Mode
  Relational Operator{,1,3,6,9,12} (6 alike) : RelationalOperator  Operator=<=  OutDataTypeStr=boolean  RndMeth=Simplest
  Relational Operator10 : RelationalOperator  OutDataTypeStr=boolean  RndMeth=Simplest
  Relational Operator11 : RelationalOperator  OutDataTypeStr=boolean  RndMeth=Simplest
  Relational Operator2 : RelationalOperator  Operator=>  OutDataTypeStr=boolean  RndMeth=Simplest
  Relational Operator4 : RelationalOperator  Operator===  OutDataTypeStr=boolean  RndMeth=Simplest
  Relational Operator5 : RelationalOperator  Operator=>  OutDataTypeStr=boolean  RndMeth=Simplest
  Relational Operator7 : RelationalOperator  Operator===  OutDataTypeStr=boolean  RndMeth=Simplest
  Relational Operator8 : RelationalOperator  Operator===  OutDataTypeStr=boolean  RndMeth=Simplest
  Relay1 : Relay  OnSwitchValue=KTQD_OPDHoldGradeUp_Deg  OffSwitchValue=KTQD_OPDHoldGradeDown_Deg  OutDataTypeStr=boolean
  SR_Latch{,1..4} (5 alike) : hcu_lib/Basic_Blocks/SR_Latch
  Saturation Dynamic{,1..4} (5 alike) : simulink/Discontinuities/Saturation Dynamic  OutMin=[]  OutMax=[]  OutDataTypeStr=Inherit: Same as second input  OutDataType=fixdt(1, 16)  OutScaling=2^-10  DoSatur=off
  Switch{,6..12} (8 alike) : Switch  Criteria=u2 > Threshold
  Switch3 : Switch  Criteria=u2 ~= 0
  Switch4 : Switch  Criteria=u2 ~= 0
  Switch5 : Switch  Criteria=u2 ~= 0
  Triggered Subsystem : Subsystem  TreatAsAtomicUnit=on
  Unit Delay : UnitDelay  SampleTime=-1  HasFrameUpgradeWarning=on
  VTQD_PedalMapWhlTq_Nm : Outport
  VTQD_EVDriveModeValid_flg : Outport  Port=2
  VTQD_RegenTqLimitEn_flg : Outport  Port=3
  VTQD_PedAccTqEn_flg : Outport  Port=4
  VTQD_SlideRegenLimTq_Nm : Outport  Port=5
  wires:
  LHM/1(VTQD_PedalMapWhlTqLHM_Nm) -> Merge/1
  [VTQD_EVDriveMode_enum] -> NoLHM/7(VTQD_EVDriveMode_enum)
  [VTQD_GearActualPosn_enum] -> NoLHM/6(VTQD_GearActualPosn_enum)
  GearShiftCheck/2 -> NoLHM/Action
  GearShiftCheck/1 -> LHM/Action
  Logical Operator1/1 -> Logical Operator/2
  [VTQD_EVDriveModeValid_flg] -> Logical Operator1/1
  Logical Operator/1 -> GearShiftCheck/1
  Constant2/1 -> Switch/3  "VTQD_EVDriveModeValid_flg"
  [VTQD_RollingShaftSpd_rpm] -> NoLHM/5(VTQD_RollingShaftSpd_rpm)
  [VTQD_RollRegenEnable_flg] -> NoLHM/4(VTQD_RollRegenEnable_flg)
  VTQD_RollingShaftSpd_rpm/1 -> [VTQD_RollingShaftSpd_rpm]
  VTQD_RollRegenEnable_flg/1 -> [VTQD_RollRegenEnable_flg]
  VTQD_RegenMode_enum/1 -> [VTQD_RegenMode_enum]
  VTQD_ActAPSPosn_pct/1 -> [VTQD_ActAPSPosn_pct]
  VTQD_EVDriveMode_enum/1 -> [VTQD_EVDriveMode_enum]
  VTQD_LimpHomeAct_flg/1 -> [VTQD_LimpHomeAct_flg]
  VTQD_GearActualPosn_enum/1 -> [VTQD_GearActualPosn_enum]
  VTQD_TqTargetShaftSpd_rpm/1 -> [VTQD_TqTargetShaftSpd_rpm]
  [VTQD_TqTargetShaftSpd_rpm] -> NoLHM/2(VTQD_TqTargetShaftSpd_rpm)
  [VTQD_RegenMode_enum] -> NoLHM/3(VTQD_RegenMode_enum)
  [VTQD_ActAPSPosn_pct] -> NoLHM/1(VTQD_ActAPSPosn_pct)
  [VTQD_ActAPSPosn_pct] -> LHM/1(VTQD_ActAPSPosn_pct)
  [VTQD_TqTargetShaftSpd_rpm] -> LHM/2(VTQD_TqTargetShaftSpd_rpm)
  VTQD_RollRegenDisableReq_flg/1 -> [VTQD_RollRegenDisableReq_flg]
  VINP_HSAActive_flg/1 -> [VINP_HSAActive_flg]
  Switch5/1 -> [VTQD_GRADE_Deg]  "VTQD_GRADE_Deg"
  Constant4/1 -> Switch5/2
  Constant13/1 -> Switch5/1
  Switch3/1 -> Switch4/3
  [VTQD_TqTargetShaftSpd_rpm] -> Abs/1
  Constant5/1 -> Saturation Dynamic/3
  SR_Latch/1 -> AND/1
  Relational Operator/1 -> AND/2, NOT/1
  Constant10/1 -> Relational Operator/2
  Constant12/1 -> Saturation Dynamic1/3
  Saturation Dynamic1/1 -> Switch4/1
  Saturation Dynamic/1 -> Switch3/1
  Abs/1 -> Relational Operator/1
  Abs1/1 -> MTQD_PedalMapClimbUpLim_Z_Nm/2
  [VTQD_TqTargetShaftSpd_rpm] -> Abs1/1
  AND/1 -> Switch3/2  "VTQD_ActHSAActive_flg"
  [VTQD_GRADE_Deg] -> MTQD_PedalMapClimbUpLim_Z_Nm/1
  NOT/1 -> SR_Latch/2
  MTQD_PedalMapClimbUpLim_Z_Nm/1 -> Saturation Dynamic/1  "VTQD_PedalMapClimbUpLim_Nm"
  Constant11/1 -> Saturation Dynamic1/1
  VVMC_ADASActive_flg/1 -> [VVMC_ADASActive_flg]
  Logical Operator2/1 -> Switch4/2
  Saturation Dynamic2/1 -> Switch3/3
  Constant14/1 -> Saturation Dynamic2/1
  VVMC_ActMaxSlideRate_pct/1 -> [VVMC_ActMaxSlideRate_pct]
  VVMC_LongAcc_Gps/1 -> [VVMC_LongAcc_Gps]
  VVMC_EstSlope_Deg/1 -> [VVMC_EstSlope_Deg]
  [VVMC_EstSlope_Deg] -> Switch5/3
  Constant21/1 -> AND2/2
  [VTQD_SlideRegenLimTq_Nm] -> Switch8/1
  [VTQD_RegenTqLimitEn_flg] -> AND2/1
  AND2/1 -> Switch8/2
  Add1/1 -> Saturation Dynamic4/2
  Detect Decrease/1 -> AND1/1
  Switch6/1 -> Add1/2
  [VVMC_LongAcc_Gps] -> "MTQD_SlideRegenTqGain_Z_Nm "/2
  Relational Operator2/1 -> SR_Latch1/2
  Constant18/1 -> Switch6/3
  Constant20/1 -> Relational Operator2/2
  [VTQD_RollRegenDisableReq_flg] -> Detect Decrease/1
  Add/1 -> Saturation Dynamic3/2
  Delay/1 -> [VTQD_LastSlideRegenLimTq_Nm]  "VTQD_LastSlideRegenLimTq_Nm"
  [VTQD_OrigPedalMapWhlTq_Nm] -> Relational Operator2/1
  Constant19/1 -> Relational Operator1/2
  SR_Latch1/1 -> VTQD_RegenTqLimitEn_flg/1, [VTQD_RegenTqLimitEn_flg], Switch6/2  "VTQD_RegenTqLimitEn_flg"
  "MTQD_SlideRegenTqGain_Z_Nm "/1 -> Add1/1  "VTQD_SlideRegenLimTqGain_Nm"
  Constant17/1 -> Saturation Dynamic3/3
  Constant23/1 -> Saturation Dynamic4/3
  [VVMC_ActMaxSlideRate_pct] -> Add/1
  [VTQD_OrigPedalMapWhlTq_Nm] -> Relational Operator1/1
  Relational Operator1/1 -> AND1/2
  Saturation Dynamic3/1 -> "MTQD_SlideRegenTqGain_Z_Nm "/1  "VTQD_SlideRateDev_pct"
  Saturation Dynamic4/1 -> Delay/1, VTQD_SlideRegenLimTq_Nm/1, [VTQD_SlideRegenLimTq_Nm]  "VTQD_SlideRegenLimTq_Nm"
  Constant15/1 -> Add/2
  Constant22/1 -> Saturation Dynamic4/1
  Constant16/1 -> Saturation Dynamic3/1
  AND1/1 -> SR_Latch1/1
  [VTQD_LastSlideRegenLimTq_Nm] -> Switch6/1
  VINP_RrPTCSActive_flg/1 -> [VINP_RrPTCSActive_flg]
  VINP_BrkPedalPos_pct/1 -> [VINP_BrkPedalPos_pct]
  VTQD_LowIdleAccPedal_flg/1 -> [VTQD_LowIdleAccPedal_flg]
  VINP_VehSpeed_kph/1 -> [VINP_VehSpeed_kph]
  VTQD_BrkSwSta_flg/1 -> [VTQD_BrkSwSta_flg]
  VINP_ADASACCSta_enum/1 -> [VINP_ADASACCSta_enum]
  VTQR_NoABSREDUWhlTqReq_Nm/1 -> [VTQR_NoABSREDUWhlTqReq_Nm]
  VTQR_NoABSFEDUWhlTqReq_Nm/1 -> [VTQR_NoABSFEDUWhlTqReq_Nm]
  VINP_FrPTCSActive_flg/1 -> [VINP_FrPTCSActive_flg]
  VPMM_PwrSta_enum/1 -> [VPMM_PwrSta_enum]
  VINP_SWCResUpSta_flg/1 -> [VINP_SWCResUpSta_flg]
  task_time_s/1 -> [task_time_s]
  VTQD_CreepPrLoadEnable_flg/1 -> [VTQD_CreepPrLoadEnable_flg]
  VTQD_SysMode_enum/1 -> [VTQD_SysMode_enum]
  Equal/1 -> Detect Increase/1
  [VINP_FrPTCSActive_flg] -> Logical Operator3/2
  Logical Operator3/1 -> AND3/1
  AND3/1 -> SR_Latch3/1
  [VTQD_BrkSwSta_flg] -> OR/2
  Detect Increase/1 -> AND3/2
  NOT1/1 -> OR/1
  [VTQD_LowIdleAccPedal_flg] -> NOT1/1
  Constant25/1 -> Equal/2
  SR_Latch3/1 -> [VTQD_ADASShutOff_flg]  "VTQD_ADASShutOff_flg"
  OR/1 -> SR_Latch3/2
  [VINP_RrPTCSActive_flg] -> Logical Operator3/1
  [VVMC_ADASActive_flg] -> Logical Operator2/3
  [VTQD_RollRegenDisableReq_flg] -> Logical Operator2/2
  [VTQD_ADASShutOff_flg] -> Logical Operator2/1
  Max/1 -> [VTQD_OrigPedTqLowLim_Nm]  "VTQD_OrigPedTqLowLim_Nm"
  [VTQD_BrkRgnLatchTqLim_Nm] -> Max/2
  Switch8/1 -> Max/1
  [VTQD_OrigPedTqLowLim_Nm] -> Saturation Dynamic2/3
  [VTQD_SlideTqLowLim_Nm] -> Switch9/3
  [VTQR_NoABSFEDUWhlTqReq_Nm] -> Add2/2
  Constant27/1 -> Relational Operator6/2
  Constant24/1 -> Relational Operator3/2
  Switch9/1 -> [VTQD_BrkRgnLatchTqLim_Nm]  "VTQD_BrkRgnLatchTqLim_Nm"
  Constant26/1 -> Relational Operator5/2
  Min/1 -> Switch9/1
  [VINP_BrkPedalPos_pct] -> Relational Operator3/1
  Relational Operator6/1 -> AND4/2
  [VVMC_EstSlope_Deg] -> Relational Operator6/1
  [VTQR_NoABSREDUWhlTqReq_Nm] -> Add2/1
  AND4/1 -> SR_Latch2/1
  Switch10/1 -> Min/1, Delay2/1
  Relational Operator5/1 -> AND4/1
  Constant28/1 -> Min/2
  Delay2/1 -> Switch10/1
  [VINP_BrkPedalPos_pct] -> Relational Operator5/1
  Add2/1 -> Switch10/3
  [VINP_ADASACCSta_enum] -> Equal/1
  Switch7/1 -> VTQD_PedalMapWhlTq_Nm/1  "VTQD_PedalMapWhlTq_Nm"
  [VINP_HSAActive_flg] -> OR1/2
  OR1/1 -> SR_Latch/1
  VTQD_OPDHoldEnRel_flg/1 -> [VTQD_OPDHoldEnRel_flg]
  Delay1/1 -> OR1/1
  [VVMC_ActMaxSlideRate_pct] -> MTQD_OrigPedTqLowLim_Z_Nm/1
  [VINP_YawRate_degps] -> Abs2/1
  [VVMC_ActStESCYaw_degps] -> Add4/2
  Abs2/1 -> Add4/1
  Add4/1 -> MTQD_YawTqLowLim_Y_Nm/1  "VTQD_TqLowLimYawDev_degps"
  MTQD_OrigPedTqLowLim_Z_Nm/1 -> [VTQD_SlideTqLowLim_Nm], Max1/1  "VTQD_SlideTqLowLim_Nm"
  MTQD_YawTqLowLim_Y_Nm/1 -> Max1/2  "VTQD_YawTqLowLim_Nm"
  Max1/1 -> [VTQD_PreDecTqLowLim_Nm]  "VTQD_PreDecTqLowLim_Nm"
  [VTQD_PreDecTqLowLim_Nm] -> Switch8/3
  VINP_SASAngle_Deg/1 -> [VINP_SASAngle_Deg]
  VVMC_ActStESCYaw_degps/1 -> [VVMC_ActStESCYaw_degps]
  VINP_YawRate_degps/1 -> [VINP_YawRate_degps]
  Abs3/1 -> MTQD_OrigPedTqLowLim_Z_Nm/2
  [VINP_SASAngle_Deg] -> Abs3/1
  [VTQD_OPDHoldEnRel_flg] -> Delay1/1
  [VVMC_EstSlope_Deg] -> NoLHM/8(VVMC_EstSlope_Deg)
  [VTQD_APSReqTimer_s] -> NoLHM/9(VTQD_APSReqTimer_s)
  VTQD_APSReqTimer_s/1 -> [VTQD_APSReqTimer_s]
  [VTQD_LowIdleAccPedal_flg] -> NoLHM/10(VTQD_LowIdleAccPedal_flg)
  [VINP_ADASACCSta_enum] -> Unit Delay/1
  Constant72/1 -> Relational Operator4/2
  Unit Delay/1 -> Relational Operator4/1
  [VINP_ADASACCSta_enum] -> Relational Operator7/1
  Constant29/1 -> Relational Operator7/2
  Relational Operator7/1 -> OR2/1
  Relational Operator4/1 -> AND5/1
  AND5/1 -> Detect Increase1/1, SR_Latch4/1
  Constant30/1 -> Relational Operator8/2
  [VINP_ADASACCSta_enum] -> Relational Operator8/1
  Relational Operator8/1 -> OR2/2
  OR2/1 -> AND5/2
  SR_Latch4/1 -> [VTQD_ACCCancelDet_flg]  "VTQD_ACCCancelDet_flg"
  [VTQD_ACCCancelDet_flg] -> AND6/1
  Switch11/1 -> Switch7/1
  Switch4/1 -> Switch7/3, Max2/1, Max3/1, Relational Operator11/1  "VTQD_ActPedalMapWhlTq_Nm"
  [VTQD_ActAPSPosn_pct] -> Relational Operator9/1
  Relational Operator9/1 -> OR3/1
  Constant31/1 -> Relational Operator9/2
  Constant32/1 -> AND5/3
  Detect Increase1/1 -> Triggered Subsystem/Trigger
  VVMC_LastADASWhlTqReq_Nm/1 -> Triggered Subsystem/1(in1)
  Triggered Subsystem/1(Out1) -> [VTQD_ACCCancelMemTq_Nm]  "VTQD_ACCCancelMemTq_Nm"
  [VTQD_ActAPSPosn_pct] -> Triggered Subsystem/2(In2)
  Triggered Subsystem/2(Out2) -> [VTQD_ACCCancelMemPosn_pct]  "VTQD_ACCCancelMemPosn_pct"
  [VTQD_ActAPSPosn_pct] -> Relational Operator10/1
  [VTQD_ACCCancelMemPosn_pct] -> Relational Operator10/2
  [VTQD_ACCCancelMemTq_Nm] -> Max2/2
  Relational Operator10/1 -> Switch11/2
  Max2/1 -> Switch11/1
  [VTQD_ActAPSPosn_pct] -> Add13/1
  [VTQD_ACCCancelMemPosn_pct] -> Add13/2
  Constant69/1 -> Divide7/2
  Add13/1 -> Divide7/1
  Divide7/1 -> Add3/2
  [VTQD_ACCCancelMemTq_Nm] -> Add3/1
  Max3/1 -> Switch11/3
  Add3/1 -> Max3/2
  [VTQD_ACCCancelMemTq_Nm] -> Relational Operator11/2
  Relational Operator11/1 -> OR3/2
  OR3/1 -> SR_Latch4/2
  AND6/1 -> Switch7/2
  Constant33/1 -> AND6/2
  [VTQD_OPDHoldEnRel_flg] -> NoLHM/11(VTQD_OPDHoldEnRel_flg)
  [VTQD_OPDHoldActRelTq_Nm] -> NoLHM/12(VTQD_OPDHoldActRelTq_Nm)
  [VTQD_VehActSpd_kph] -> NoLHM/13(VTQD_VehActSpd_kph)
  VTQD_OPDHoldActRelTq_Nm/1 -> [VTQD_OPDHoldActRelTq_Nm]
  VTQD_VehActSpd_kph/1 -> [VTQD_VehActSpd_kph]
  [VVMC_EstSlope_Deg] -> Relay1/1
  Relay1/1 -> [VTQD_SlopeUp_flg]  "VTQD_SlopeUp_flg"
  [VTQD_SlopeUp_flg] -> NoLHM/14(VTQD_SlopeUp_flg)
  VINP_IVISnowModeCmd_flg/1 -> [VINP_IVISnowModeCmd_flg]
  [VINP_IVISnowModeCmd_flg] -> NoLHM/15(VINP_IVISnowModeCmd_flg)
  [task_time_s] -> Pedal G-Control Mode/6(task_time_s)
  [VTQD_SysMode_enum] -> Pedal G-Control Mode/1(VINP_SCPSystemMode_enum)
  [VINP_BrkPedalPos_pct] -> Pedal G-Control Mode/12(VINP_BrkPedalPos_pct)
  [VTQD_CreepPrLoadEnable_flg] -> Pedal G-Control Mode/11(VTQD_CreepPrLoadEnable_flg)
  [VTQD_ActAPSPosn_pct] -> Pedal G-Control Mode/7(VTQD_ActAPSPosn_pct)
  [VTQD_TqTargetShaftSpd_rpm] -> Pedal G-Control Mode/8(VTQD_TqTargetShaftSpd_rpm)
  Pedal G-Control Mode/1(VTQD_PedAccTqEn_flg) -> VTQD_PedAccTqEn_flg/1, [VTQD_PedAccTqEn_flg]
  Pedal G-Control Mode/2(VTQD_PedalTqCal_Nm) -> [VTQD_PedalTqCal_Nm]
  Constant34/1 -> Pedal G-Control Mode/16(VINP_IVICreepOnSW_flg)  "VTQD_IVICreepOnSW_flg"
  Constant8/1 -> Pedal G-Control Mode/14(VVMC_SmartRegenReq_mps2)  "VTQD_SmartRegenReq_mps2"
  [VVMC_LongAcc_Gps] -> Pedal G-Control Mode/9(VVMC_LongAcc_Gps)
  [VINP_VehSpeed_kph] -> Pedal G-Control Mode/10(VINP_VehSpeed_kph)
  [VTQD_RegenMode_enum] -> Pedal G-Control Mode/4(VTQD_RegenMode_enum)
  [VTQD_APSReqTimer_s] -> Pedal G-Control Mode/17(VTQD_APSReqTimer_s)
  [VINP_SWC2RCustomizeSta_flg] -> Pedal G-Control Mode/5(VINP_SWC2RCustomizeSta_flg)
  [VTQD_GearActualPosn_enum] -> Pedal G-Control Mode/3(VTQD_GearActualPosn_enum)
  Constant9/1 -> Pedal G-Control Mode/15(VINP_IVISmartRegenSW_flg)  "VTQD_IVISmartRegenSW_flg"
  [VPMM_PwrSta_enum] -> Pedal G-Control Mode/2(VPMM_PwrSta_enum)
  Constant7/1 -> Pedal G-Control Mode/13(VINP_IVIPedalGRegenLim_pct)  "VTQD_IVIPedalGRegenLim_pct"
  Constant6/1 -> Switch/1
  Constant3/1 -> Switch/2
  Switch/1 -> VTQD_EVDriveModeValid_flg/1, [VTQD_EVDriveModeValid_flg]  "VTQD_EVDriveModeValid_flg"
  Merge/1 -> Switch12/3
  [VTQD_PedalTqCal_Nm] -> Switch12/1
  [VTQD_PedAccTqEn_flg] -> Switch12/2
  Switch12/1 -> Saturation Dynamic2/2, Saturation Dynamic/2, Saturation Dynamic1/2, [VTQD_OrigPedalMapWhlTq_Nm]  "VTQD_OrigPedalMapWhlTq_Nm"
  Relational Operator12/1 -> AND7/2
  Constant1/1 -> Relational Operator12/2
  Relational Operator3/1 -> AND7/1
  AND7/1 -> SR_Latch2/2
  [VTQD_VehActSpd_kph] -> Relational Operator12/1
  SR_Latch2/1 -> Switch9/2, Switch10/2  "VTQD_BrkRgnLatchEn_flg"
  NoLHM/1(VTQD_PedalMapWhlTqNoLHM_Nm) -> Merge/2
  [VTQD_PreDecTqLowLim_Nm] -> NoLHM/17(VTQD_PreDecTqLowLim_Nm)
  [VTQD_IVIRockModeEn_flg] -> NoLHM/16(VTQD_IVIRockModeEn_flg)
  VTQD_IVIRockModeEn_flg/1 -> [VTQD_IVIRockModeEn_flg]
  [VTQD_BrkSwSta_flg] -> NoLHM/18(VTQD_BrkSwSta_flg)
  [VTQD_CreepEnable_flg] -> NoLHM/19(VTQD_CreepEnable_flg)
  VTQD_CreepEnable_flg/1 -> [VTQD_CreepEnable_flg]
  [VINP_SWCResUpSta_flg] -> Pedal G-Control Mode/18(VINP_SWCResUpSta_flg)
  VINP_SWC2RCustomizeSta_flg/1 -> [VINP_SWC2RCustomizeSta_flg]
  VDDM_VehMalfunLevel_enum/1 -> [VDDM_VehMalfunLevel_enum]
  [VTQD_GearActualPosn_enum] -> LHM/3(VTQD_GearActualPosn_enum)
  [VDDM_VehMalfunLevel_enum] -> LHM/4(VDDM_VehMalfunLevel_enum)
  [VVMC_EstSlope_Deg] -> LHM/5(VVMC_EstSlope_Deg)
  [VTQD_VehActSpd_kph] -> LHM/6(VTQD_VehActSpd_kph)
  Constant99/1 -> Logical Operator18/2
  [VTQD_LimpHomeAct_flg] -> Logical Operator18/1
  Logical Operator18/1 -> Logical Operator/1

== system tqd/TQD/TorqueDemand/TorqueModule/DriverWhlTqDem/RollingRegenJudge ==
  VDHP_LowIdleAccPedal_flg : Inport
  VINP_VehSpd_kph : Inport  Port=2
  VTQD_TqTargetShaftSpd_rpm : Inport  Port=3
  VTQD_RollRegenDisableReq_flg : Inport  Port=4
  VTQD_TqSourceFr_enum : Inport  Port=5
  VTQD_TqSourceRr_enum : Inport  Port=6
  VTQD_CreepEnable_flg : Inport  Port=7
  Constant : Constant  Value=ENUM_TQSOURCE_CC
  Constant1 : Constant  Value=ENUM_TQSOURCE_ADAS
  Constant2 : Constant  Value=ENUM_TQSOURCE_APS
  Constant3 : Constant  Value=ENUM_TQSOURCE_CC
  Constant4 : Constant  Value=ENUM_TQSOURCE_ADAS
  Constant5 : Constant  Value=ENUM_TQSOURCE_APS
  Detect Increase : simulink/Logic and Bit Operations/Detect Increase  vinit=0.0  OutDataTypeStr=boolean
  Equal{,1..5} (6 alike) : RelationalOperator  Operator===  OutDataTypeStr=boolean  RndMeth=Simplest
  Logical Operator : Logic  Inputs=5  AllPortsSameDT=off  OutDataTypeStr=boolean
  Logical Operator1 : Logic  Operator=NOT  AllPortsSameDT=off  OutDataTypeStr=boolean
  Logical Operator10 : Logic  Operator=OR  AllPortsSameDT=off  OutDataTypeStr=boolean
  Logical Operator11 : Logic  Operator=NOT  AllPortsSameDT=off  OutDataTypeStr=boolean
  Logical Operator12 : Logic  Operator=NOT  AllPortsSameDT=off  OutDataTypeStr=boolean
  Logical Operator5 : Logic  Operator=OR  Inputs=3  AllPortsSameDT=off  OutDataTypeStr=boolean
  Logical Operator9 : Logic  Operator=OR  Inputs=3  AllPortsSameDT=off  OutDataTypeStr=boolean
  Relay : Relay  OnSwitchValue=KTQD_RegenOnSpd_kph  OffSwitchValue=KTQD_RegenOffSpd_kph
      settings: AttributesFormatString=|
      | ON: %<OnSwitchValue>
      | OFF: %<OffSwitchValue>
  Switch2 : Switch  Criteria=u2 ~= 0
      settings: AttributesFormatString=<%<Criteria>>
  Unit Delay : UnitDelay  SampleTime=-1  HasFrameUpgradeWarning=on
  Unit Delay1 : UnitDelay  SampleTime=-1  HasFrameUpgradeWarning=on
  VTQD_RollRegenEnable_flg : Outport
  VTQD_RollingShaftSpd_rpm : Outport  Port=2
  wires:
  Equal5/1 -> Logical Operator9/3
  Equal3/1 -> Logical Operator9/1
  Equal4/1 -> Logical Operator9/2
  Constant4/1 -> Equal4/2
  [VTQD_TqSourceRr_enum] -> Equal4/1
  Constant5/1 -> Equal5/2
  [VTQD_TqSourceRr_enum] -> Equal5/1
  Constant3/1 -> Equal3/2
  [VTQD_TqSourceRr_enum] -> Equal3/1
  Constant2/1 -> Equal2/2
  [VTQD_TqSourceFr_enum] -> Equal2/1
  Constant1/1 -> Equal1/2
  [VTQD_TqSourceFr_enum] -> Equal1/1
  Constant/1 -> Equal/2
  Logical Operator11/1 -> Logical Operator/5
  Logical Operator10/1 -> Logical Operator11/1
  Logical Operator9/1 -> Logical Operator10/2
  Logical Operator5/1 -> Logical Operator10/1
  [VTQD_CreepEnable_flg] -> Unit Delay1/1
  Equal2/1 -> Logical Operator5/3
  Equal1/1 -> Logical Operator5/2
  Equal/1 -> Logical Operator5/1
  VTQD_CreepEnable_flg/1 -> [VTQD_CreepEnable_flg]
  VTQD_TqSourceFr_enum/1 -> [VTQD_TqSourceFr_enum]
  VTQD_TqSourceRr_enum/1 -> [VTQD_TqSourceRr_enum]
  [VTQD_RollRegenDisableReq_flg] -> Logical Operator1/1
  VTQD_RollRegenDisableReq_flg/1 -> [VTQD_RollRegenDisableReq_flg]
  Unit Delay/1 -> Switch2/3
  Switch2/1 -> VTQD_RollingShaftSpd_rpm/1, Unit Delay/1  "VTQD_RollingShaftSpd_rpm"
  [VTQD_TqTargetShaftSpd_rpm] -> Switch2/1
  Detect Increase/1 -> Switch2/2
  [VTQD_RollRegenEnable_flg] -> Detect Increase/1
  VTQD_TqTargetShaftSpd_rpm/1 -> [VTQD_TqTargetShaftSpd_rpm]
  [VINP_VehSpd_kph] -> Relay/1
  VINP_VehSpd_kph/1 -> [VINP_VehSpd_kph]
  VDHP_LowIdleAccPedal_flg/1 -> [VTQD_LowIdleAccPedal_flg]
  Logical Operator/1 -> VTQD_RollRegenEnable_flg/1, [VTQD_RollRegenEnable_flg]  "VTQD_RollRegenEnable_flg"
  Unit Delay1/1 -> Logical Operator12/1
  Relay/1 -> Logical Operator/2
  Logical Operator12/1 -> Logical Operator/4
  Logical Operator1/1 -> Logical Operator/3
  [VTQD_LowIdleAccPedal_flg] -> Logical Operator/1
  [VTQD_TqSourceFr_enum] -> Equal/1
